simulink model "Single_Axis_Roll_Disturbance_Est_Feedback"  (R2024b)
settings: Solver=ode4  StartTime=0.0  StopTime=0.2  FixedStep=0.001  RelTol=1e-3
undefined symbols (not defined in the file): Ad_pitch, Ad_roll, Ad_yaw, Bd_pitch, Bd_roll, Bd_yaw, Cd_pitch, Cd_roll, Cd_yaw, K_pitch, K_roll, K_yaw
libraries: simulink x6
settings Model: Creator=Zohaib  LastModifiedBy=Zohaib
settings DataIOCC: ReturnWorkspaceOutputs=off

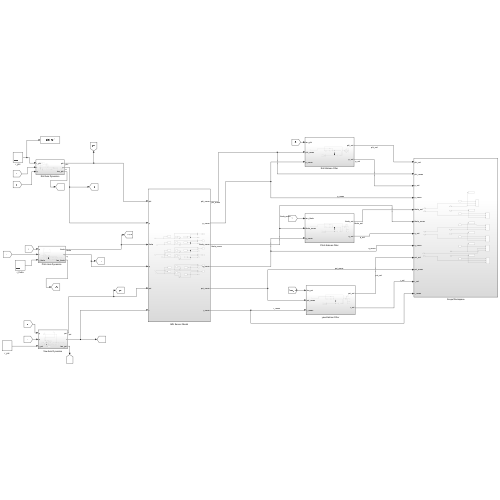
[thumbnail: Simulink's stored preview of the top-level diagram]
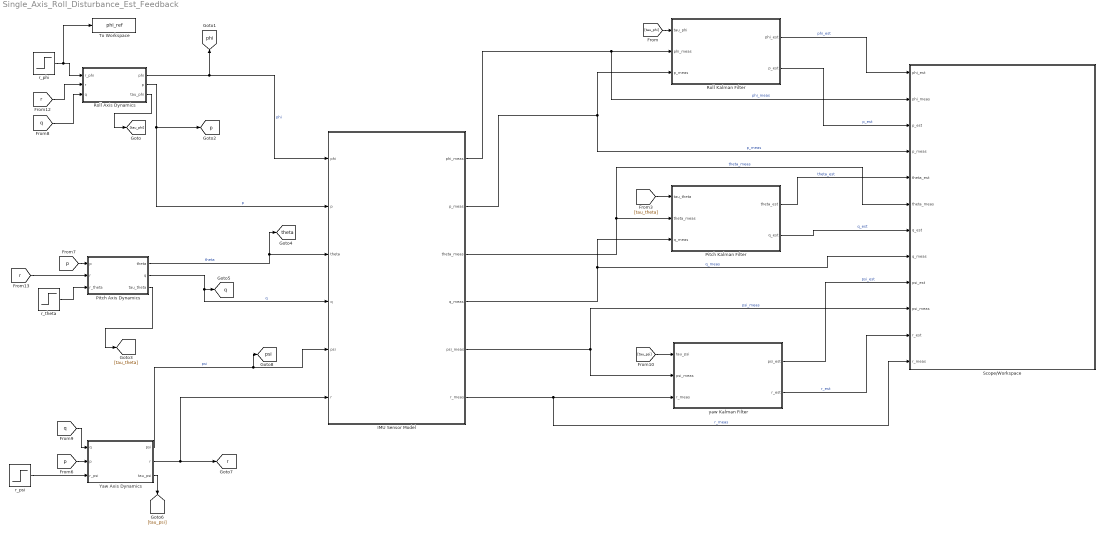
== system Single_Axis_Roll_Disturbance_Est_Feedback ==
  IMU Sensor Model : Subsystem
  Pitch Axis Dynamics : Subsystem
  Pitch Kalman Filter : Subsystem
  Roll Axis Dynamics : Subsystem
  Roll Kalman Filter : Subsystem
  Scope/Workspace : Subsystem
  To Workspace : ToWorkspace  VariableName=phi_ref  SaveFormat=Timeseries  SampleTime=-1
  Yaw Axis Dynamics : Subsystem
  r_phi : Step  Time=0  After=5*(pi/180)  SampleTime=0.001
  r_psi : Step  Time=0  After=0  SampleTime=0
  r_theta : Step  Time=0  After=0  SampleTime=0
  yaw Kalman Filter : Subsystem
  tag scope: p=global, phi=global, psi=global, q=global, r=global, theta=global
  wires:
  yaw Kalman Filter/2(r_est) -> Scope/Workspace/11(r_est)  "r_est"
  IMU Sensor Model/5(psi_meas) -> yaw Kalman Filter/2(psi_meas), Scope/Workspace/10(psi_meas)  "psi_meas"
  Yaw Axis Dynamics/2(r) -> [r], IMU Sensor Model/6(r)
  Yaw Axis Dynamics/3(tau_psi) -> [tau_psi]
  IMU Sensor Model/6(r_meas) -> yaw Kalman Filter/3(r_meas), Scope/Workspace/12(r_meas)  "r_meas"
  yaw Kalman Filter/1(psi_est) -> Scope/Workspace/9(psi_est)  "psi_est"
  Pitch Axis Dynamics/3(tau_theta) -> [tau_theta]
  r_psi/1 -> Yaw Axis Dynamics/3(r_psi)
  r_theta/1 -> Pitch Axis Dynamics/3(r_theta)
  [p] -> Yaw Axis Dynamics/2(p)
  [r] -> Roll Axis Dynamics/2(r)
  Roll Axis Dynamics/1(phi) -> [phi], IMU Sensor Model/1(phi)  "phi"
  [tau_theta] -> Pitch Kalman Filter/1(tau_theta)
  [r] -> Pitch Axis Dynamics/2(r)
  Pitch Kalman Filter/1(theta_est) -> Scope/Workspace/5(theta_est)  "theta_est"
  [p] -> Pitch Axis Dynamics/1(p)
  IMU Sensor Model/4(q_meas) -> Pitch Kalman Filter/3(q_meas), Scope/Workspace/8(q_meas)  "q_meas"
  [tau_phi] -> Roll Kalman Filter/1(tau_phi)
  [q] -> Roll Axis Dynamics/3(q)
  Roll Axis Dynamics/3(tau_phi) -> [tau_phi]
  [tau_psi] -> yaw Kalman Filter/1(tau_psi)
  r_phi/1 -> To Workspace/1, Roll Axis Dynamics/1(r_phi)
  IMU Sensor Model/2(p_meas) -> Roll Kalman Filter/3(p_meas), Scope/Workspace/4(p_meas)  "p_meas"
  [q] -> Yaw Axis Dynamics/1(q)
  IMU Sensor Model/1(phi_meas) -> Scope/Workspace/2(phi_meas), Roll Kalman Filter/2(phi_meas)  "phi_meas"
  Pitch Axis Dynamics/1(theta) -> [theta], IMU Sensor Model/3(theta)  "theta"
  Roll Kalman Filter/1(phi_est) -> Scope/Workspace/1(phi_est)  "phi_est"
  Yaw Axis Dynamics/1(psi) -> [psi], IMU Sensor Model/5(psi)  "psi"
  Pitch Kalman Filter/2(q_est) -> Scope/Workspace/7(q_est)  "q_est"
  IMU Sensor Model/3(theta_meas) -> Scope/Workspace/6(theta_meas), Pitch Kalman Filter/2(theta_meas)  "theta_meas"
  Roll Kalman Filter/2(p_est) -> Scope/Workspace/3(p_est)  "p_est"
  Roll Axis Dynamics/2(p) -> [p], IMU Sensor Model/2(p)  "p"
  Pitch Axis Dynamics/2(q) -> [q], IMU Sensor Model/4(q)  "q"

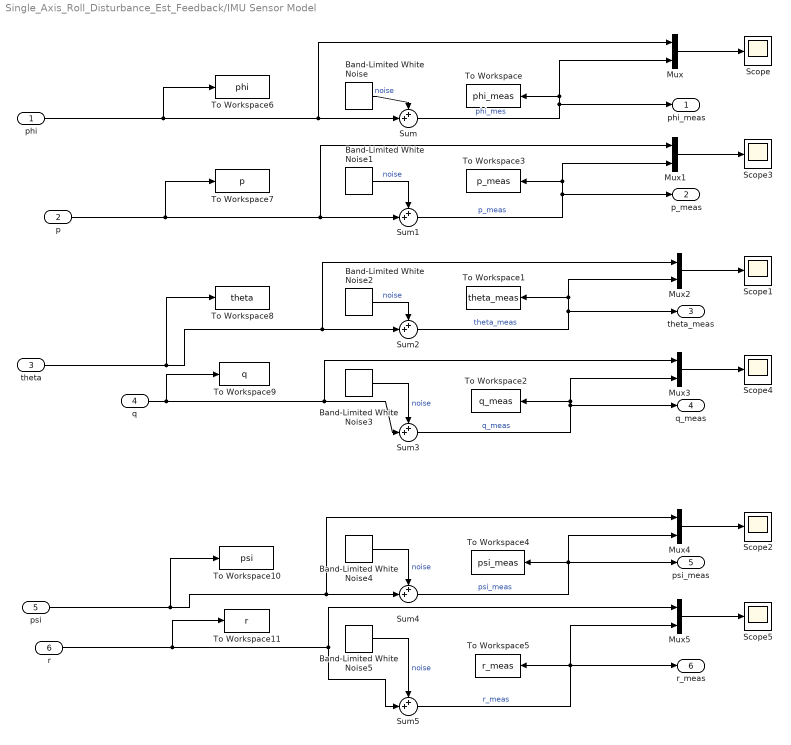
== system Single_Axis_Roll_Disturbance_Est_Feedback/IMU Sensor Model ==
  phi : Inport
  p : Inport  Port=2
  theta : Inport  Port=3
  q : Inport  Port=4
  psi : Inport  Port=5
  r : Inport  Port=6
  Band-Limited White Noise : simulink/Sources/Band-Limited White Noise  Cov=7.16e-7  Ts=0.001  seed=1
  Band-Limited White Noise1 : simulink/Sources/Band-Limited White Noise  Cov=1.69e-6  Ts=0.001  seed=4
  Band-Limited White Noise2 : simulink/Sources/Band-Limited White Noise  Cov=7.16e-7  Ts=0.001  seed=2
  Band-Limited White Noise3 : simulink/Sources/Band-Limited White Noise  Cov=1.69e-6  Ts=0.001  seed=5
  Band-Limited White Noise4 : simulink/Sources/Band-Limited White Noise  Cov=7.16e-7  Ts=0.001  seed=3
  Band-Limited White Noise5 : simulink/Sources/Band-Limited White Noise  Cov=1.69e-6  Ts=0.001  seed=6
  Mux{,1..5} (6 alike) : Mux  Inputs=2
  Scope{,1..5} (6 alike) : Scope
  Sum{,1..5} (6 alike) : Sum  Inputs=++|
  To Workspace : ToWorkspace  VariableName=phi_meas  SaveFormat=Timeseries  SampleTime=-1
  To Workspace1 : ToWorkspace  VariableName=theta_meas  SaveFormat=Timeseries  SampleTime=-1
  To Workspace10 : ToWorkspace  VariableName=psi  SaveFormat=Timeseries  SampleTime=-1
  To Workspace11 : ToWorkspace  VariableName=r  SaveFormat=Timeseries  SampleTime=-1
  To Workspace2 : ToWorkspace  VariableName=q_meas  SaveFormat=Timeseries  SampleTime=-1
  To Workspace3 : ToWorkspace  VariableName=p_meas  SaveFormat=Timeseries  SampleTime=-1
  To Workspace4 : ToWorkspace  VariableName=psi_meas  SaveFormat=Timeseries  SampleTime=-1
  To Workspace5 : ToWorkspace  VariableName=r_meas  SaveFormat=Timeseries  SampleTime=-1
  To Workspace6 : ToWorkspace  VariableName=phi  SaveFormat=Timeseries  SampleTime=-1
  To Workspace7 : ToWorkspace  VariableName=p  SaveFormat=Timeseries  SampleTime=-1
  To Workspace8 : ToWorkspace  VariableName=theta  SaveFormat=Timeseries  SampleTime=-1
  To Workspace9 : ToWorkspace  VariableName=q  SaveFormat=Timeseries  SampleTime=-1
  phi_meas : Outport
  p_meas : Outport  Port=2
  theta_meas : Outport  Port=3
  q_meas : Outport  Port=4
  psi_meas : Outport  Port=5
  r_meas : Outport  Port=6
  wires:
  Band-Limited White Noise1/1 -> Sum1/1  "noise"
  Band-Limited White Noise3/1 -> Sum3/1  "noise"
  Sum3/1 -> q_meas/1, Mux3/2, To Workspace2/1  "q_meas"
  Sum2/1 -> theta_meas/1, Mux2/2, To Workspace1/1  "theta_meas"
  psi/1 -> To Workspace10/1, Mux4/1, Sum4/2
  Band-Limited White Noise4/1 -> Sum4/1  "noise"
  phi/1 -> To Workspace6/1, Sum/2, Mux/1
  Sum4/1 -> psi_meas/1, Mux4/2, To Workspace4/1  "psi_meas"
  Band-Limited White Noise2/1 -> Sum2/1  "noise"
  q/1 -> To Workspace9/1, Mux3/1, Sum3/2
  Mux/1 -> Scope/1
  Sum1/1 -> p_meas/1, Mux1/2, To Workspace3/1  "p_meas"
  p/1 -> To Workspace7/1, Sum1/2, Mux1/1
  Band-Limited White Noise/1 -> Sum/1  "noise"
  Sum/1 -> phi_meas/1, To Workspace/1, Mux/2  "phi_mes"
  Mux2/1 -> Scope1/1
  Sum5/1 -> To Workspace5/1, r_meas/1, Mux5/2  "r_meas"
  Band-Limited White Noise5/1 -> Sum5/1  "noise"
  Mux3/1 -> Scope4/1
  Mux1/1 -> Scope3/1
  Mux4/1 -> Scope2/1
  theta/1 -> To Workspace8/1, Mux2/1, Sum2/2
  Mux5/1 -> Scope5/1
  r/1 -> To Workspace11/1, Sum5/2, Mux5/1

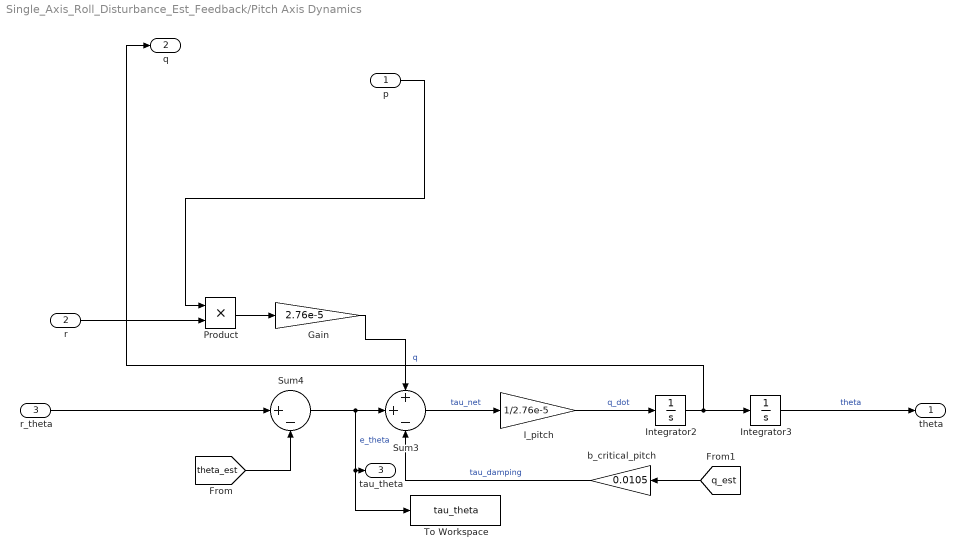
== system Single_Axis_Roll_Disturbance_Est_Feedback/Pitch Axis Dynamics ==
  p : Inport
  r : Inport  Port=2
  r_theta : Inport  Port=3
  Gain : Gain  Gain=2.76e-5
  I_pitch : Gain  Gain=1/2.76e-5
  Integrator2 : Integrator
  Integrator3 : Integrator
  Product : Product
  Sum3 : Sum  Inputs=++-
  Sum4 : Sum  Inputs=|+-
  To Workspace : ToWorkspace  VariableName=tau_theta  SaveFormat=Timeseries  SampleTime=-1
  b_critical_pitch : Gain  Gain=0.0105
  theta : Outport
  q : Outport  Port=2
  tau_theta : Outport  Port=3
  wires:
  r/1 -> Product/2
  Integrator2/1 -> q/1, Integrator3/1  "q"
  b_critical_pitch/1 -> Sum3/3  "tau_damping"
  Sum3/1 -> I_pitch/1  "tau_net"
  Product/1 -> Gain/1
  Sum4/1 -> To Workspace/1, tau_theta/1, Sum3/2  "e_theta"
  Gain/1 -> Sum3/1
  I_pitch/1 -> Integrator2/1  "q_dot"
  Integrator3/1 -> theta/1  "theta"
  p/1 -> Product/1
  r_theta/1 -> Sum4/1
  [theta_est] -> Sum4/2
  [q_est] -> b_critical_pitch/1

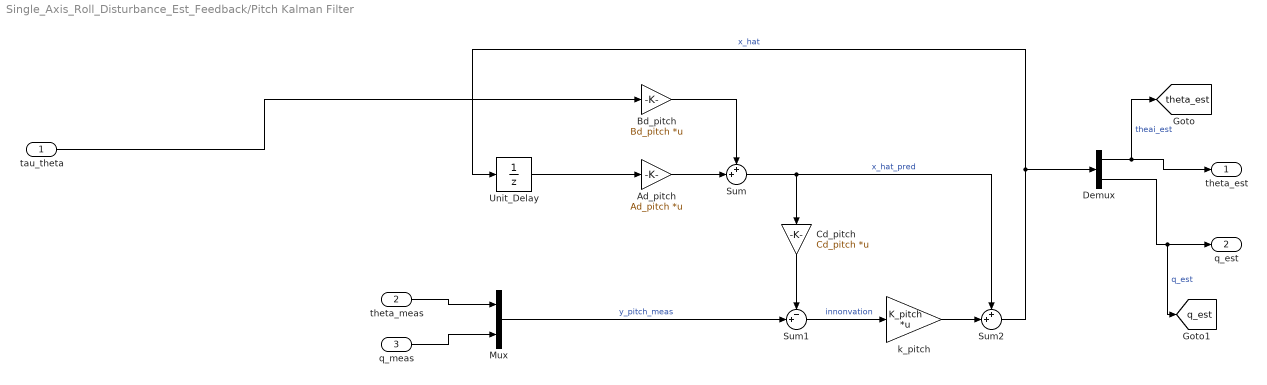
== system Single_Axis_Roll_Disturbance_Est_Feedback/Pitch Kalman Filter ==
  tau_theta : Inport
  theta_meas : Inport  Port=2
  q_meas : Inport  Port=3
  Ad_pitch : Gain  Gain=Ad_pitch  Multiplication=Matrix(K*u)
  Bd_pitch : Gain  Gain=Bd_pitch  Multiplication=Matrix(K*u)
  Cd_pitch : Gain  Gain=Cd_pitch  Multiplication=Matrix(K*u)
  Demux : Demux  Outputs=2
  Mux : Mux  Inputs=2
  Sum : Sum  Inputs=++|
  Sum1 : Sum  Inputs=-+|
  Sum2 : Sum  Inputs=++|
  Unit_Delay : UnitDelay  InitialCondition=[0;0]  SampleTime=0.001  HasFrameUpgradeWarning=on
  k_pitch : Gain  Gain=K_pitch  Multiplication=Matrix(K*u)
  theta_est : Outport
  q_est : Outport  Port=2
  tag scope: q_est=global, theta_est=global
  wires:
  Ad_pitch/1 -> Sum/2
  q_meas/1 -> Mux/2
  Bd_pitch/1 -> Sum/1
  Sum/1 -> Sum2/1, Cd_pitch/1  "x_hat_pred"
  k_pitch/1 -> Sum2/2
  Sum2/1 -> Demux/1, Unit_Delay/1  "x_hat"
  Mux/1 -> Sum1/2  "y_pitch_meas"
  theta_meas/1 -> Mux/1
  Cd_pitch/1 -> Sum1/1
  Sum1/1 -> k_pitch/1  "innonvation"
  Unit_Delay/1 -> Ad_pitch/1
  Demux/1 -> [theta_est], theta_est/1  "theai_est"
  Demux/2 -> q_est/1, [q_est]  "q_est"
  tau_theta/1 -> Bd_pitch/1

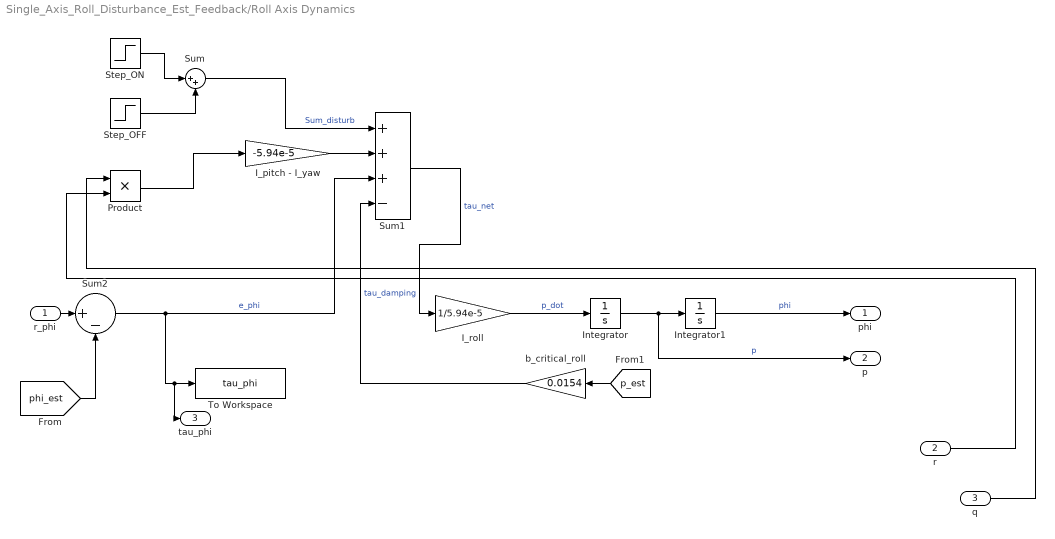
== system Single_Axis_Roll_Disturbance_Est_Feedback/Roll Axis Dynamics ==
  r_phi : Inport
  r : Inport  Port=2
  q : Inport  Port=3
  I_pitch - I_yaw : Gain  Gain=-5.94e-5
  I_roll : Gain  Gain=1/5.94e-5
  Integrator : Integrator
  Integrator1 : Integrator
  Product : Product
  Step_OFF : Step  Time=0.105  After=-0.12  SampleTime=0.001
  Step_ON : Step  Time=0.1  After=0.12  SampleTime=0.001
  Sum : Sum  Inputs=|++
  Sum1 : Sum  Inputs=+++-
  Sum2 : Sum  Inputs=|+-
  To Workspace : ToWorkspace  VariableName=tau_phi  SaveFormat=Timeseries  SampleTime=-1
  b_critical_roll : Gain  Gain=0.0154
  phi : Outport
  p : Outport  Port=2
  tau_phi : Outport  Port=3
  wires:
  Integrator1/1 -> phi/1  "phi"
  Sum2/1 -> Sum1/3, tau_phi/1, To Workspace/1  "e_phi"
  Product/1 -> I_pitch - I_yaw/1
  I_roll/1 -> Integrator/1  "p_dot"
  Integrator/1 -> p/1, Integrator1/1  "p"
  Sum1/1 -> I_roll/1  "tau_net"
  r/1 -> Product/2
  q/1 -> Product/1
  r_phi/1 -> Sum2/1
  [phi_est] -> Sum2/2
  [p_est] -> b_critical_roll/1
  b_critical_roll/1 -> Sum1/4  "tau_damping"
  I_pitch - I_yaw/1 -> Sum1/2
  Sum/1 -> Sum1/1  "Sum_disturb"
  Step_OFF/1 -> Sum/2
  Step_ON/1 -> Sum/1

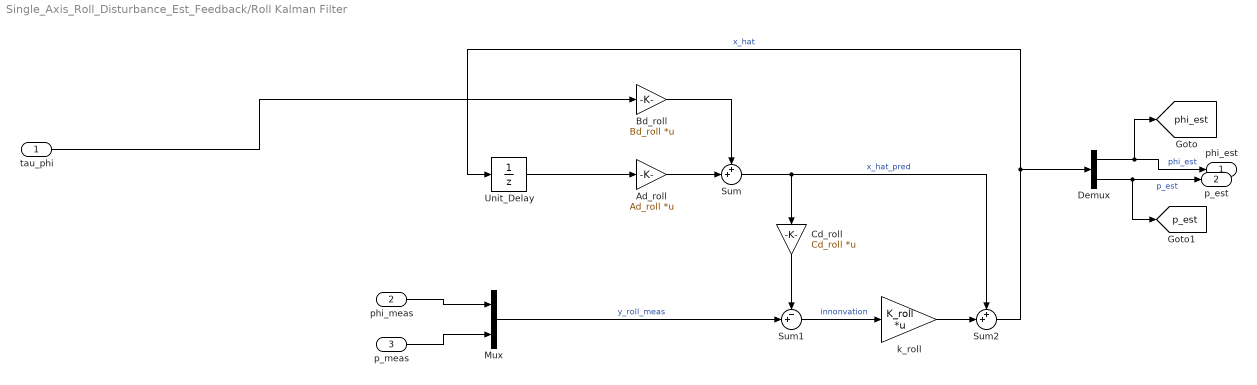
== system Single_Axis_Roll_Disturbance_Est_Feedback/Roll Kalman Filter ==
  tau_phi : Inport
  phi_meas : Inport  Port=2
  p_meas : Inport  Port=3
  Ad_roll : Gain  Gain=Ad_roll  Multiplication=Matrix(K*u)
  Bd_roll : Gain  Gain=Bd_roll  Multiplication=Matrix(K*u)
  Cd_roll : Gain  Gain=Cd_roll  Multiplication=Matrix(K*u)
  Demux : Demux  Outputs=2
  Mux : Mux  Inputs=2
  Sum : Sum  Inputs=++|
  Sum1 : Sum  Inputs=-+|
  Sum2 : Sum  Inputs=++|
  Unit_Delay : UnitDelay  InitialCondition=[0;0]  SampleTime=0.001  HasFrameUpgradeWarning=on
  k_roll : Gain  Gain=K_roll  Multiplication=Matrix(K*u)
  phi_est : Outport
  p_est : Outport  Port=2
  tag scope: p_est=global, phi_est=global
  wires:
  Ad_roll/1 -> Sum/2
  p_meas/1 -> Mux/2
  Bd_roll/1 -> Sum/1
  Sum/1 -> Sum2/1, Cd_roll/1  "x_hat_pred"
  k_roll/1 -> Sum2/2
  Sum2/1 -> Demux/1, Unit_Delay/1  "x_hat"
  Mux/1 -> Sum1/2  "y_roll_meas"
  phi_meas/1 -> Mux/1
  Cd_roll/1 -> Sum1/1
  Sum1/1 -> k_roll/1  "innonvation"
  Unit_Delay/1 -> Ad_roll/1
  Demux/1 -> [phi_est], phi_est/1  "phi_est"
  Demux/2 -> [p_est], p_est/1  "p_est"
  tau_phi/1 -> Bd_roll/1

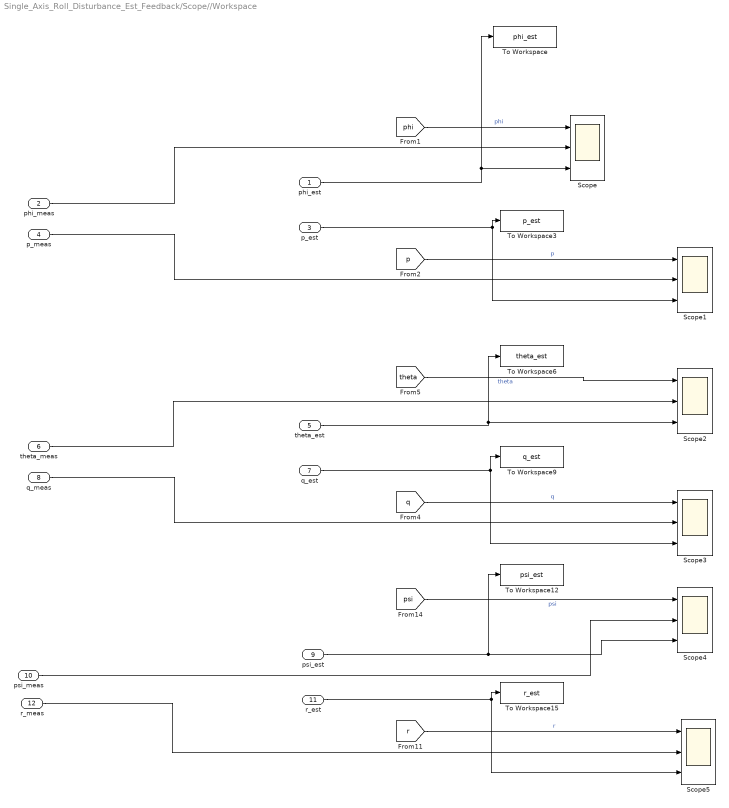
== system Single_Axis_Roll_Disturbance_Est_Feedback/Scope//Workspace ==
  phi_est : Inport
  phi_meas : Inport  Port=2
  p_est : Inport  Port=3
  p_meas : Inport  Port=4
  theta_est : Inport  Port=5
  theta_meas : Inport  Port=6
  q_est : Inport  Port=7
  q_meas : Inport  Port=8
  psi_est : Inport  Port=9
  psi_meas : Inport  Port=10
  r_est : Inport  Port=11
  r_meas : Inport  Port=12
  Scope{,1..5} (6 alike) : Scope  NumInputPorts=3
  To Workspace : ToWorkspace  VariableName=phi_est  SaveFormat=Timeseries  SampleTime=-1
  To Workspace12 : ToWorkspace  VariableName=psi_est  SaveFormat=Timeseries  SampleTime=-1
  To Workspace15 : ToWorkspace  VariableName=r_est  SaveFormat=Timeseries  SampleTime=-1
  To Workspace3 : ToWorkspace  VariableName=p_est  SaveFormat=Timeseries  SampleTime=-1
  To Workspace6 : ToWorkspace  VariableName=theta_est  SaveFormat=Timeseries  SampleTime=-1
  To Workspace9 : ToWorkspace  VariableName=q_est  SaveFormat=Timeseries  SampleTime=-1
  wires:
  [r] -> Scope5/1  "r"
  [p] -> Scope1/1  "p"
  theta_meas/1 -> Scope2/2
  [phi] -> Scope/1  "phi"
  r_est/1 -> Scope5/3, To Workspace15/1
  psi_est/1 -> To Workspace12/1, Scope4/3
  q_est/1 -> Scope3/3, To Workspace9/1
  [q] -> Scope3/1  "q"
  phi_meas/1 -> Scope/2
  psi_meas/1 -> Scope4/2
  p_meas/1 -> Scope1/2
  phi_est/1 -> To Workspace/1, Scope/3
  q_meas/1 -> Scope3/2
  theta_est/1 -> To Workspace6/1, Scope2/3
  [psi] -> Scope4/1  "psi"
  r_meas/1 -> Scope5/2
  p_est/1 -> Scope1/3, To Workspace3/1
  [theta] -> Scope2/1  "theta"

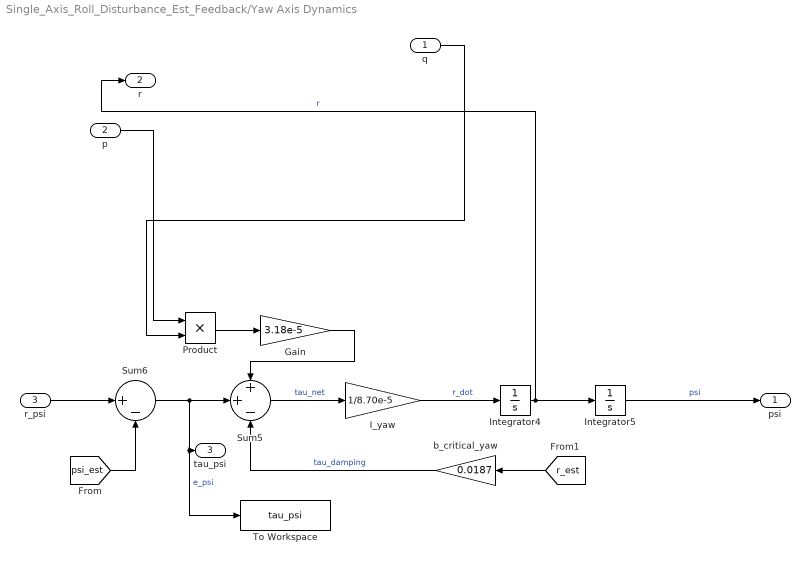
== system Single_Axis_Roll_Disturbance_Est_Feedback/Yaw Axis Dynamics ==
  q : Inport
  p : Inport  Port=2
  r_psi : Inport  Port=3
  Gain : Gain  Gain=3.18e-5
  I_yaw : Gain  Gain=1/8.70e-5
  Integrator4 : Integrator
  Integrator5 : Integrator
  Product : Product
  Sum5 : Sum  Inputs=++-
  Sum6 : Sum  Inputs=|+-
  To Workspace : ToWorkspace  VariableName=tau_psi  SaveFormat=Timeseries  SampleTime=-1
  b_critical_yaw : Gain  Gain=0.0187
  psi : Outport
  r : Outport  Port=2
  tau_psi : Outport  Port=3
  wires:
  Sum6/1 -> To Workspace/1, tau_psi/1, Sum5/2  "e_psi"
  Gain/1 -> Sum5/1
  Integrator5/1 -> psi/1  "psi"
  I_yaw/1 -> Integrator4/1  "r_dot"
  Integrator4/1 -> r/1, Integrator5/1  "r"
  q/1 -> Product/2
  b_critical_yaw/1 -> Sum5/3  "tau_damping"
  Product/1 -> Gain/1
  r_psi/1 -> Sum6/1
  p/1 -> Product/1
  Sum5/1 -> I_yaw/1  "tau_net"
  [psi_est] -> Sum6/2
  [r_est] -> b_critical_yaw/1

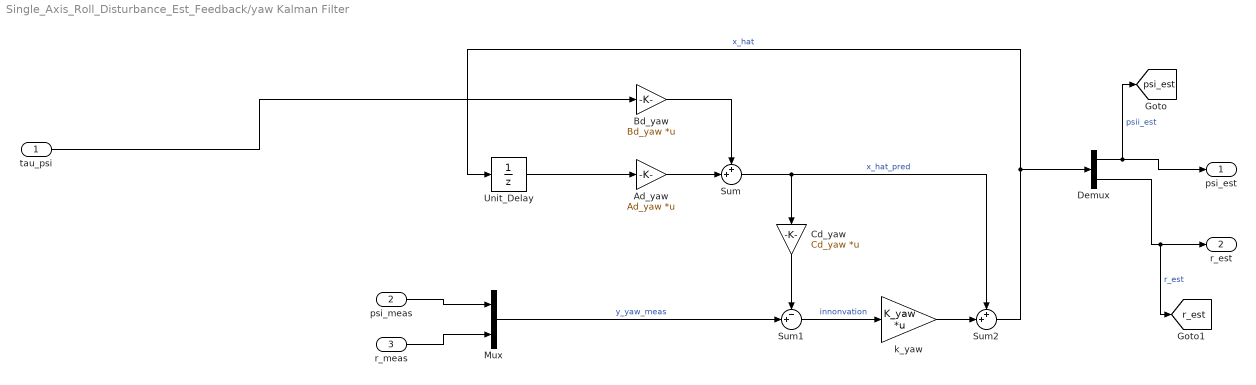
== system Single_Axis_Roll_Disturbance_Est_Feedback/yaw Kalman Filter ==
  tau_psi : Inport
  psi_meas : Inport  Port=2
  r_meas : Inport  Port=3
  Ad_yaw : Gain  Gain=Ad_yaw  Multiplication=Matrix(K*u)
  Bd_yaw : Gain  Gain=Bd_yaw  Multiplication=Matrix(K*u)
  Cd_yaw : Gain  Gain=Cd_yaw  Multiplication=Matrix(K*u)
  Demux : Demux  Outputs=2
  Mux : Mux  Inputs=2
  Sum : Sum  Inputs=++|
  Sum1 : Sum  Inputs=-+|
  Sum2 : Sum  Inputs=++|
  Unit_Delay : UnitDelay  InitialCondition=[0;0]  SampleTime=0.001  HasFrameUpgradeWarning=on
  k_yaw : Gain  Gain=K_yaw  Multiplication=Matrix(K*u)
  psi_est : Outport
  r_est : Outport  Port=2
  tag scope: psi_est=global, r_est=global
  wires:
  Ad_yaw/1 -> Sum/2
  r_meas/1 -> Mux/2
  Bd_yaw/1 -> Sum/1
  Sum/1 -> Sum2/1, Cd_yaw/1  "x_hat_pred"
  k_yaw/1 -> Sum2/2
  Sum2/1 -> Demux/1, Unit_Delay/1  "x_hat"
  Mux/1 -> Sum1/2  "y_yaw_meas"
  psi_meas/1 -> Mux/1
  Cd_yaw/1 -> Sum1/1
  Sum1/1 -> k_yaw/1  "innonvation"
  Unit_Delay/1 -> Ad_yaw/1
  Demux/1 -> [psi_est], psi_est/1  "psii_est"
  Demux/2 -> r_est/1, [r_est]  "r_est"
  tau_psi/1 -> Bd_yaw/1
